simulink model "PWM_GEN"  (R2022b)
settings: Solver=VariableStepAuto  StartTime=0.0  StopTime=10.0  RelTol=1e-3
libraries: spsMosfetLib x4, spsCurrentMeasurementLib x1, spsVoltageMeasurementLib x1
settings Model: Creator=nisha  LastModifiedBy=nisha

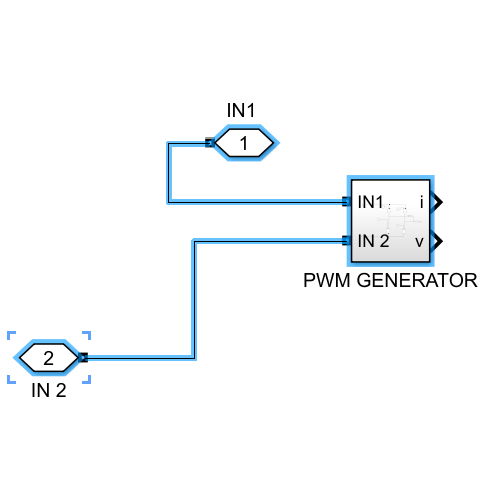
[thumbnail: Simulink's stored preview of the top-level diagram]
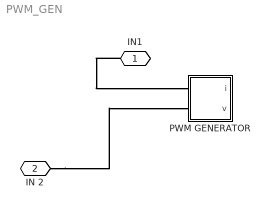
== system PWM_GEN ==
  PWM GENERATOR : Subsystem
  "IN1 " : PMIOPort  Side=Left
  IN 2 : PMIOPort  Port=2  Side=Left
  connections:
  "IN1 "/RConn1 -- PWM GENERATOR/LConn1
  IN 2/RConn1 -- PWM GENERATOR/LConn2

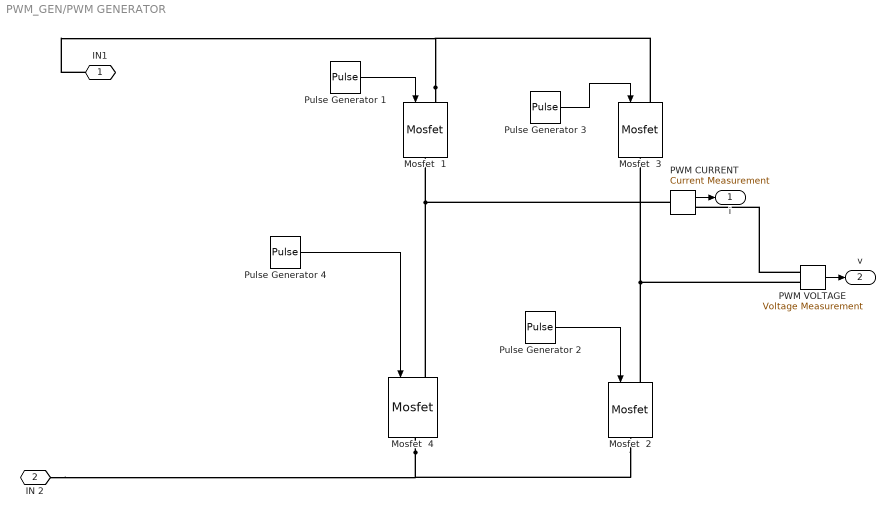
== system PWM_GEN/PWM GENERATOR ==
  Mosfet  {1..4} (4 alike) : spsMosfetLib/Mosfet  Ron=0.1  Lon=0  Rd=0.01  Vfd=0  IC=0  Rs=1e5  Cs=inf  Measurements=off
  PWM CURRENT : spsCurrentMeasurementLib/Current Measurement  PhasorSimulation=off  OutputType=Complex  PSBequivalent=0
  PWM VOLTAGE : spsVoltageMeasurementLib/Voltage Measurement  PhasorSimulation=off  OutputType=Complex  PSBequivalent=0
  Pulse Generator {1..4} (4 alike) : DiscretePulseGenerator  PulseType=Time based  Period=0.02  PulseWidth=50
  "IN1 " : PMIOPort  Side=Left
  IN 2 : PMIOPort  Port=2  Side=Left
  i : Outport
  v : Outport  Port=2
  wires:
  PWM CURRENT/1 -> i/1
  Pulse Generator 3/1 -> Mosfet  3/1
  Pulse Generator 2/1 -> Mosfet  2/1
  Pulse Generator 1/1 -> Mosfet  1/1
  Pulse Generator 4/1 -> Mosfet  4/1
  PWM VOLTAGE/1 -> v/1
  connections:
  Mosfet  4/RConn1 -- IN 2/RConn1 -- Mosfet  2/RConn1
  Mosfet  1/LConn1 -- "IN1 "/RConn1 -- Mosfet  3/LConn1
  Mosfet  2/LConn1 -- PWM VOLTAGE/LConn2 -- Mosfet  3/RConn1
  Mosfet  4/LConn1 -- PWM CURRENT/LConn1 -- Mosfet  1/RConn1
  PWM VOLTAGE/LConn1 -- PWM CURRENT/RConn1
